simulink model "Lab3_DigitalModulation"  (R2023b)
settings: Solver=FixedStepDiscrete  StartTime=0.0  StopTime=inf  FixedStep=1/fs  RelTol=1e-3
values from neighbouring files (symbols this model uses):
  binary = audioToBinary(wav, 7)    [Lab3_DigitalModulation.m]    (also in audioToBinary.m = bin2dec(char_reshaped'))
undefined symbols (not defined in the file or in its folder): fs
libraries: commdigbbndam3 x2, commchan3 x1, commsink2 x1, impairlib x1, dspsrcs4 x1
settings Model: Creator=Emilija  LastModifiedBy=minhk
settings SolverCC: AlgebraicLoopSolver=TrustRegion
settings DebuggingCC: UnconnectedInputMsg=warning  UnconnectedOutputMsg=warning  UnconnectedLineMsg=warning
settings ModelReferenceCC: EnableRefExpFcnMdlSchedulingChecks=on

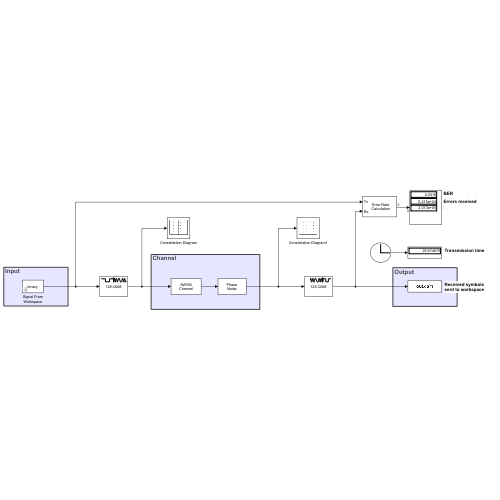
[thumbnail: Simulink's stored preview of the top-level diagram]
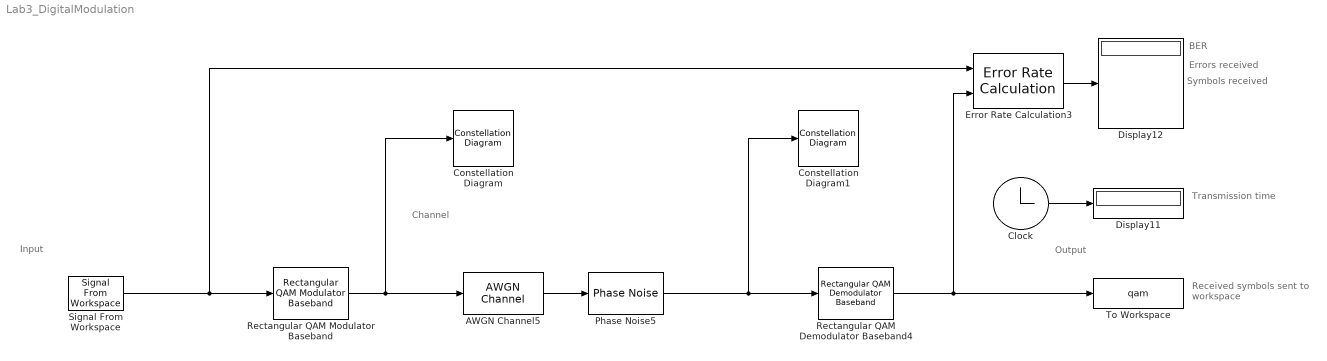
== system Lab3_DigitalModulation ==
  note: Output
  note: Errors received
  note: Symbols received
  note: BER
  note: Channel
  note: Transmission time
  note: Received symbols sent to workspace
  note: Input
  AWGN Channel5 : commchan3/AWGN Channel  LegacyMode=on  NoiseMethod="Signal to noise ratio  (SNR)"  noiseMode="Signal to noise ratio  (SNR)"  EbNo=15  EsNo=40  SNR=20  BitsPerSymbol=2  SignalPower=1  SamplesPerSymbol=1  SymbolPeriod=1e-6  VarianceSource=Parameter  Variance=1  RandomStream=Global stream  Seed=54321  SimulateUsing=Code generation
  Clock : Clock
      settings: Decimation=1000
  Constellation Diagram : ConstellationDiagram  WindowPosition=[54.000000,488.000000,410.000000,300.000000,]  Visible=on  ScopeFrameLocation=window  XLimits=[-1.5006 1.5006]  YLimits=[-1.5006 1.5006]  ColorFading=on  DefaultConfigurationName=comm.scopes.ConstellationDiagramBlockCfg
  Constellation Diagram1 : ConstellationDiagram  WindowPosition=[56.000000,96.000000,410.000000,300.000000,]  Visible=on  ScopeFrameLocation=window  XLimits=[-1.5006 1.5006]  YLimits=[-1.5006 1.5006]  ColorFading=on  DefaultConfigurationName=comm.scopes.ConstellationDiagramBlockCfg
  Display11 : Display
      settings: Decimation=1000
  Display12 : Display
  Error Rate Calculation3 : commsink2/Error Rate Calculation  N=0  st_delay=0  cp_mode=Entire frame  subframe=[]  PMode=Port  WsName=ErrorVec  RsMode2=off  stop=on  numErr=inf  maxBits=length(binary)
  Phase Noise5 : impairlib/Phase Noise  Level=-70  FrequencyOffset=1000  SampleRate=2.1e3  RandomStream=mt19937ar with seed  Seed=2137  SimulateUsing=Interpreted execution
  Rectangular QAM Demodulator Baseband4 : commdigbbndam3/Rectangular QAM Demodulator Baseband  M=128  OutType=Integer  DecType=Hard decision  VarSource=Dialog  Variance=1  Dec=Binary  Mapping=[0:15]  PowType=Average Power  MinDist=2  AvgPow=1  PeakPow=1  Ph=0  outDtype1=Inherit via internal rule  outDtype2=Inherit via internal rule  derotateFactorWordLen=16  derotateFactorDataTypeStr=Inherit: Same word length as input  derotateFactorLastDataTypeStr=Inherit: Same word length as input  denormFactorWordLen=16  denormFactorDataTypeStr=Inherit: Same word length as input  denormFactorLastDataTypeStr=Inherit: Same word length as input  prodOutWordLen=32  prodOutOverflowMode=Wrap  prodOutRoundingMode=Floor  prodOutOvFlMode=off  prodOutOvFlModeLastStrValue=off  sumWordLen=32
  Rectangular QAM Modulator Baseband : commdigbbndam3/Rectangular QAM Modulator Baseband  M=128  InType=Integer  Enc=Binary  Mapping=[0:15]  PowType=Average Power  MinDist=2  AvgPow=1  PeakPow=1  Ph=0  outDtype=double  outWordLen=16  outUDDataType=sfix(16)  outFracLenMode=Best precision  outFracLen=15  outDataTypeStr=double  outLastDataTypeStr=double
  Signal From Workspace : dspsrcs4/Signal From Workspace  X=binary  Ts=1/fs  nsamps=1  OutputAfterFinalValue=Cyclic repetition  ignoreOrWarnInputAndFrameLengths=off  OutputFrames=off
  To Workspace : ToWorkspace  VariableName=qam  SampleTime=-1
      settings: Save2DSignal=2-D array (concatenate along first dimension)
  wires:
  Clock/1 -> Display11/1
  Rectangular QAM Demodulator Baseband4/1 -> Error Rate Calculation3/2, To Workspace/1
  Error Rate Calculation3/1 -> Display12/1
  AWGN Channel5/1 -> Phase Noise5/1
  Phase Noise5/1 -> Rectangular QAM Demodulator Baseband4/1, Constellation Diagram1/1
  Signal From Workspace/1 -> Error Rate Calculation3/1, Rectangular QAM Modulator Baseband/1
  Rectangular QAM Modulator Baseband/1 -> AWGN Channel5/1, Constellation Diagram/1
